simulink model "OneCar"  (R2017a)
settings: Solver=VariableStepAuto  StartTime=0.0  StopTime=100.0  RelTol=1e-3
settings Model: Creator=Carapinha  LastModifiedBy=Carapinha

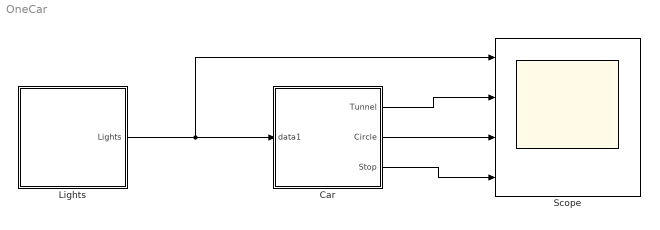
== system OneCar ==
  Car : Stateflow chart  TreatAsAtomicUnit=on
  Lights : Stateflow chart  TreatAsAtomicUnit=on
  Scope : Scope  NumInputPorts=4
  wires:
  Lights/1(Lights) -> Scope/1, Car/1(data1)
  Car/1(Tunnel) -> Scope/2
  Car/2(Circle) -> Scope/3
  Car/3(Stop) -> Scope/4

== stateflow chart OneCar/Car ==
  state Tunnel
    entry:
    Circle = 0;
    Tunnel = 1;
    Stop = 0;
  state Lights
    entry:
    Circle = 0;
    Tunnel = 0;
    Stop = 1;
  state Circle
    entry:
    Circle = 1;
    Tunnel = 0;
    Stop = 0;
  (default) -> Lights
  Lights -> Tunnel [order 1] : [data1 == 1]
  Lights -> Lights [order 2] : [data1 == 0]
  Circle -> Lights : [after(3,sec)]
  Tunnel -> Circle : [after(3,sec)]
  data: Tunnel output; data1 input; Circle output; Stop output

== stateflow chart OneCar/Lights ==
  state Red
    entry:
    Lights = 0;
  state Green
    entry:
    Lights = 1;
  (default) -> Red
  Green -> Red : [after(10, sec)]
  Red -> Green : [after(10,sec)]
  data: Lights output
